simulink model "iot_device"  (R2021a)
settings: Solver=FixedStepDiscrete  StartTime=0.0  StopTime=10.0  FixedStep=0.1  RelTol=1e-3  EnableMultiTasking=on
settings Model: Creator=WISDOM  LastModifiedBy=WISDOM
settings SolverCC: AlgebraicLoopSolver=TrustRegion  AutoInsertRateTranBlk=on
settings DataIOCC: LimitDataPoints=on
settings OptimizationCC: DefaultParameterBehavior=Inlined  EnhancedBackFolding=on  PassReuseOutputArgsAs=Individual arguments  ZeroExternalMemoryAtStartup=off  ZeroInternalMemoryAtStartup=off  OptimizeBlockOrder=speed  DifferentSizesBufferReuse=on  OptimizationCustomize=off  EfficientTunableParamExpr=on
settings DebuggingCC: ParameterTunabilityLossMsg=error  AllowSymbolicDim=off  SFUnexpectedBacktrackingDiag=warning  SFNoUnconditionalDefaultTransitionDiag=warning  SFExecutionAtInitializationDiag=none  ArithmeticOperatorsInVariantConditions=warning
settings SFSimCC: SimUseLocalCustomCode=off  MATLABDynamicMemAlloc=off  CustomCodeUndefinedFunction=UseInterfaceOnly
settings RTWCC: SystemTargetFile=ert.tlc  TemplateMakefile=ert_default_tmf  RTWUseLocalCustomCode=off
settings CodeAppCC: ForceParamTrailComments=on  IgnoreCustomStorageClasses=off  OperatorAnnotations=on  SimulinkDataObjDesc=on  SFDataObjDesc=on  InsertBlockDesc=on
settings ERTTargetCC: GenerateSampleERTMain=on  InlinedParameterPlacement=NonHierarchical  ERTCustomFileTemplate=example_file_process.tlc
settings ConfigComp: CovMetricSettings=dw  CovSaveCumulativeToWorkspaceVar=on  CovSaveSingleToWorkspaceVar=on  CovExternalEMLEnable=off  CovSFcnEnable=off

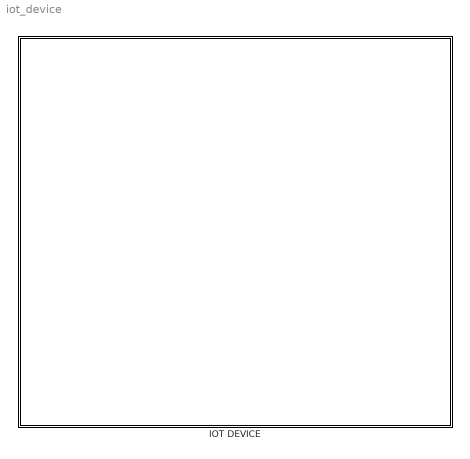
== system iot_device ==
  IOT DEVICE : Stateflow chart  TreatAsAtomicUnit=on

== stateflow chart iot_device/IOT DEVICE ==
  state gear_logic
    on every(0.05,sec): %do nothing
    state IOT
      widgets();
    (default) -> IOT
  (default) -> gear_logic : {}
  data: app local
  function widgets:
    | function widgets()
    |     %active = app.sfxLogic.getActiveStates;
    |     
    |     % turn all lights off
    |     app.GrowLightLamp.Enable = 'off';
    |     app.WaterPumpLamp.Enable = 'off';
    |     app.HumidifierLamp.Enable = 'off';
    |     app.FanLamp.Enable = 'off';
    |     
    |     if app.Light_value.Value < 20
    |         app.GrowLightLamp.Enable = 'on';
    |         app.GrowLightLamp.Color = [1.00 0.00 0.00];
    |     else
    |         app.GrowLightLamp.Enable = 'on';
    |         app.GrowLightLamp.Color = [0.00 1.00 0.00];
    |     end
    |   
    |     if app.Soil_value.Value < 40
    |         app.WaterPumpLamp.Enable = 'on';
    |         app.WaterPumpLamp.Color = [1.00 0.00 0.00];
    |     else
    |         app.WaterPumpLamp.Enable = 'on';
    |         app.WaterPumpLamp.Color = [0.00 1.00 0.00];
    |     end
    |     
    |     if app.Humidity_value.Value < 80
    |         app.HumidifierLamp.Enable = 'on';
    |         app.HumidifierLamp.Color = [1.00 0.00 0.00];
    |     else
    |         app.HumidifierLamp.Enable = 'on';
    |         app.HumidifierLamp.Color = [0.00 1.00 0.00];
    |     end
    |     
    |     if app.Temperature_value.Value < 31
    |         app.FanLamp.Enable = 'on';
    |         app.FanLamp.Color = [1.00 0.00 0.00];
    |     else
    |         app.FanLamp.Enable = 'on';
    |         app.FanLamp.Color = [0.00 1.00 0.00];
    |     end
    |     
    |     
    |     % turn gear light on and set tachometer coefficients
    |     %{
    |     switch n
    |         case 1
    |             rev = interp1([0 10],[0.5 6.5],speed,'pchip','extrap');
    |             app.FirstLamp.Enable = 'on';
    |         case 2
    |             rev = interp1([5 10 30],[0.5 1 6.5],speed,'pchip','extrap');
    |             app.SecondLamp.Enable = 'on';
    |         case 3
    |             rev = interp1([25 30 50],[0.5 1 6.5],speed,'pchip','extrap');
    |             app.ThirdLamp.Enable = 'on';
    |         case 4
    |             rev = interp1([40 50 100],[0.5 1 7],speed,'pchip','extrap');
    |             app.FourthLamp.Enable = 'on';
    |     end
    |     %}
    |     % set ui gauge values
    |     %app.SpeedometerGauge.Value = app.Soil_value.Value;
    |     %app.TachometerGauge.Value = rev;
    |     
    | end
